simulink model "VehicleModel"  (R2020b)
settings: Solver=FixedStepAuto  StartTime=0.0  StopTime=1068  FixedStep=0.1  RelTol=1e-3
model workspace (MAT data in the model file):
  t = mpt.Parameter
  t.Value = 0
  t.DataType = 'auto'
  t.Dimensions = [1 1]
(part 1 of 5)
settings Model: Creator=User  LastModifiedBy=User

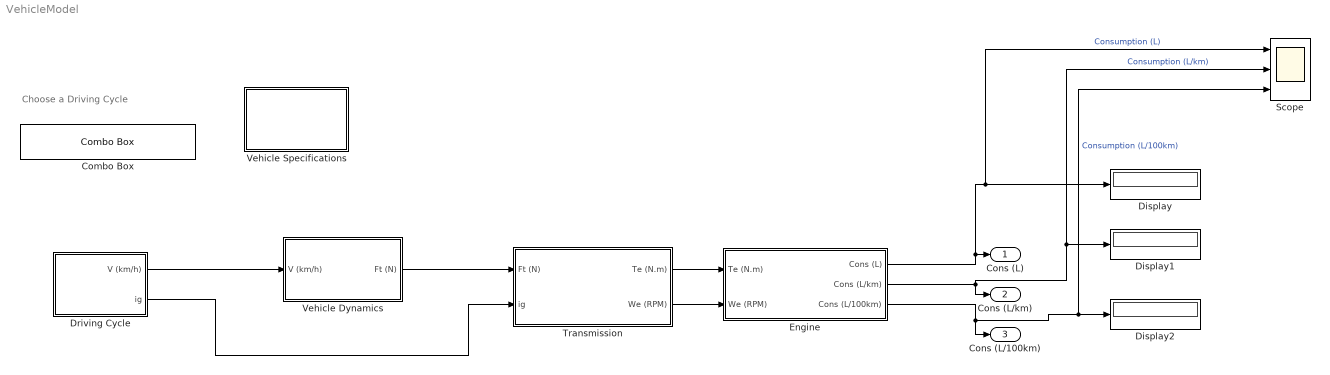
== system VehicleModel ==
  note: Choose a Driving Cycle
  Combo Box : ComboBox  LabelPosition=Hide  SelectedLabel=Highway
      settings: Values={{'Highway', 'Rural Road', 'Urban'}, [0 1 2]}
  Display : Display
  Display1 : Display
  Display2 : Display
  Driving Cycle : Subsystem
  Engine : Subsystem
  Scope : Scope  NumInputPorts=3
  Transmission : Subsystem
  Vehicle Dynamics : Subsystem
  Vehicle Specifications : Subsystem  mask{M=1320, g=9.81, rho=1.2, Af=2, Cx=0.3, rd=0.3, i0=3, ng=0.95, nd=0.97, dF=0.74, IdCon=1, IdSp=700}
      mask prompts: M "Vehicle Mass (kg)"; g "gravity (m/s2)"; rho "Air Density (kg/m3)"; Af "Surface Area (m2)"; Cx "Drag Coefficient"; rd "Dynamic Radius (m)"; i0 "Differential Gear Ratio"; ng "Gear Efficiency"; nd "Differential Efficiency"; dF "Fuel Density (kg/L)"; IdCon "Idle Consumption (L/h)"; IdSp "Idle Speed (RPM)"
  Cons (L) : Outport
  Cons (L/km) : Outport  Port=2
  Cons (L/100km) : Outport  Port=3
  wires:
  Vehicle Dynamics/1(Ft (N)) -> Transmission/1(Ft (N))
  Engine/1(Cons (L)) -> Scope/1, Display/1, Cons (L)/1  "Consumption (L)"
  Transmission/1(Te (N.m)) -> Engine/1(Te (N.m))
  Transmission/2(We (RPM)) -> Engine/2(We (RPM))
  Driving Cycle/1(" V (km/h)") -> Vehicle Dynamics/1(V (km/h))
  Engine/2(Cons (L/km)) -> Cons (L/km)/1, Scope/2, Display1/1  "Consumption (L/km)"
  Engine/3(Cons (L/100km)) -> Cons (L/100km)/1, Scope/3, Display2/1  "Consumption (L/100km)"
  Driving Cycle/2(ig) -> Transmission/2(ig)

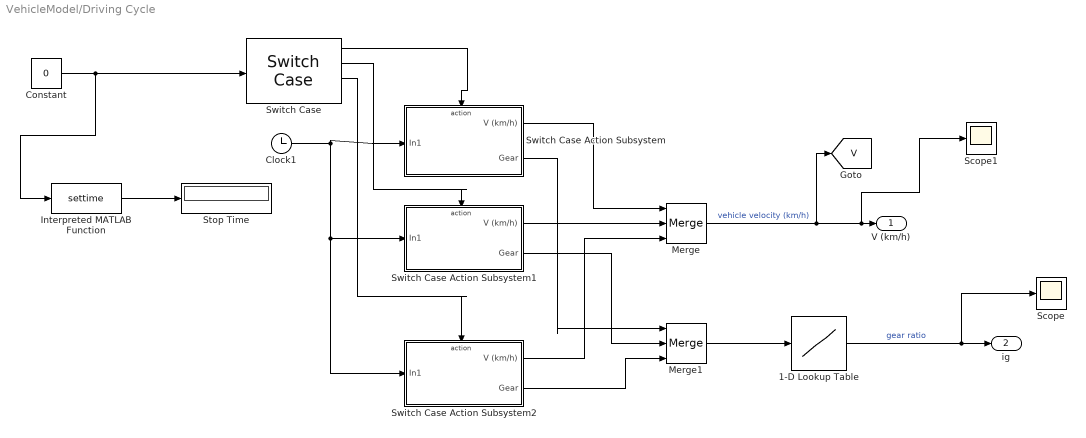
== system VehicleModel/Driving Cycle ==
  1-D Lookup Table : Lookup_n-D  NumberOfTableDimensions=1  BreakpointsForDimension1=[0 1 2 3 4 5]  Table=[0 3.5 2.31 1.52 1 0.66]  InternalRulePriority=Speed  RndMeth=Simplest  InputSameDT=on
  Clock1 : Clock
  Constant : Constant  Value=0
  Interpreted MATLAB Function : MATLABFcn  MATLABFcn=settime
  Merge : Merge  Inputs=3
  Merge1 : Merge  Inputs=3
  Scope : Scope
  Scope1 : Scope
  Stop Time : Display
  Switch Case : SwitchCase  CaseConditions={[0],[1],[2]}
  Switch Case Action Subsystem : Subsystem  TreatAsAtomicUnit=on
  Switch Case Action Subsystem1 : Subsystem  TreatAsAtomicUnit=on
  Switch Case Action Subsystem2 : Subsystem  TreatAsAtomicUnit=on
  " V (km/h)" : Outport
  ig : Outport  Port=2
  tag scope: V=global
  wires:
  1-D Lookup Table/1 -> Scope/1, ig/1  "gear ratio"
  Switch Case/1 -> Switch Case Action Subsystem/Action
  Clock1/1 -> Switch Case Action Subsystem/1(In1), Switch Case Action Subsystem1/1(In1), Switch Case Action Subsystem2/1(In1)
  Switch Case/2 -> Switch Case Action Subsystem1/Action
  Switch Case Action Subsystem1/1(V (km/h)) -> Merge/2
  Switch Case Action Subsystem/1(" V (km/h)") -> Merge/1
  Switch Case Action Subsystem/2(" Gear") -> Merge1/1
  Switch Case Action Subsystem1/2(Gear) -> Merge1/2
  Switch Case/3 -> Switch Case Action Subsystem2/Action
  Switch Case Action Subsystem2/1(V (km/h)) -> Merge/3
  Switch Case Action Subsystem2/2(Gear) -> Merge1/3
  Merge1/1 -> 1-D Lookup Table/1
  Merge/1 -> [V], Scope1/1, " V (km/h)"/1  "vehicle velocity (km/h)"
  Constant/1 -> Interpreted MATLAB Function/1, Switch Case/1
  Interpreted MATLAB Function/1 -> Stop Time/1

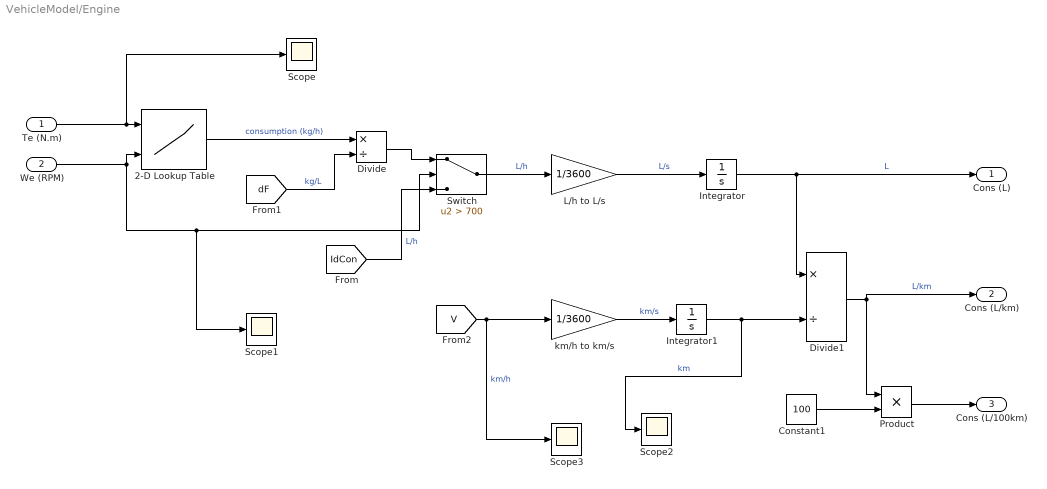
== system VehicleModel/Engine ==
  Te (N.m) : Inport
  We (RPM) : Inport  Port=2
  2-D Lookup Table : Lookup_n-D  BreakpointsForDimension1=|  BreakpointsForDimension2="[500\t1000\t1500\t2000\t2500\t3000\t3500\t4000\t4500\t5000\t5500\t6000]"  Table=|  InternalRulePriority=Speed  RndMeth=Simplest  InputSameDT=on
      BreakpointsForDimension1=|
      | [15.6
      | 31.2
      | 46.8
      | 62.4
      | 78
      | 93.6
      | 109.2
      | 124.8
      | 140.4
      | 156
      | 171.6]
      Table=|
      | [0.50	1.00	1.50	1.94	2.28	2.56	2.68	3.41	3.97	5.59	6.79	7.41;
      | 0.72	1.32	1.99	2.59	3.12	3.58	3.89	4.66	5.77	7.53	9.19	10.37;
      | 0.91	1.65	2.54	3.28	3.93	4.58	4.94	6.22	7.75	9.26	11.35	12.70;
      | 1.08	2.01	3.00	3.93	4.65	5.47	6.42	7.95	9.32	10.88	13.13	14.68;
      | 1.25	2.32	3.44	4.50	5.44	6.44	7.92	9.23	10.78	12.50	14.72	16.41;
      | 1.53	2.81	3.86	5.08	6.04	7.52	9.18	10.80	12.31	13.94	15.91	18.42;
      | 1.73	3.23	4.37	5.60	7.00	8.52	10.37	12.02	13.99	16.20	18.79	20.50;
      | 2.12	3.72	4.83	6.40	8.00	9.60	11.36	13.27	15.88	18.23	21.22	23.15;
      | 2.12	4.23	5.56	7.30	9.00	10.80	12.78	15.46	18.05	20.80	23.58	25.72;
      | 2.35	4.70	7.06	8.59	10.44	12.70	15.03	17.41	20.25	23.23	26.04	28.23;
      | 2.59	5.18	7.76	10.35	12.94	15.53	18.11	20.70	23.29	25.88	28.46	31.05]
      settings: InputPortMap=u0,u1
  Constant1 : Constant  Value=100
  Divide : Product  Inputs=*/
  Divide1 : Product  Inputs=*/
  Integrator : Integrator
  Integrator1 : Integrator
  L/h to L/s : Gain  Gain=1/3600
  Product : Product
  Scope{,1..3} (4 alike) : Scope
  Switch : Switch  Criteria=u2 > Threshold  Threshold=700
  km/h to km/s : Gain  Gain=1/3600
  Cons (L) : Outport
  Cons (L/km) : Outport  Port=2
  Cons (L/100km) : Outport  Port=3
  wires:
  Te (N.m)/1 -> Scope/1, 2-D Lookup Table/1
  Switch/1 -> L/h to L/s/1  "L/h"
  We (RPM)/1 -> 2-D Lookup Table/2, Scope1/1, Switch/2
  [dF] -> Divide/2  "kg/L"
  2-D Lookup Table/1 -> Divide/1  "consumption (kg/h)"
  L/h to L/s/1 -> Integrator/1  "L/s"
  [IdCon] -> Switch/3  "L/h"
  Integrator/1 -> Divide1/1, Cons (L)/1  "L"
  Divide/1 -> Switch/1
  [V] -> Scope3/1, km/h to km/s/1  "km/h"
  km/h to km/s/1 -> Integrator1/1  "km/s"
  Divide1/1 -> Cons (L/km)/1, Product/1  "L/km"
  Constant1/1 -> Product/2
  Product/1 -> Cons (L/100km)/1
  Integrator1/1 -> Scope2/1, Divide1/2  "km"

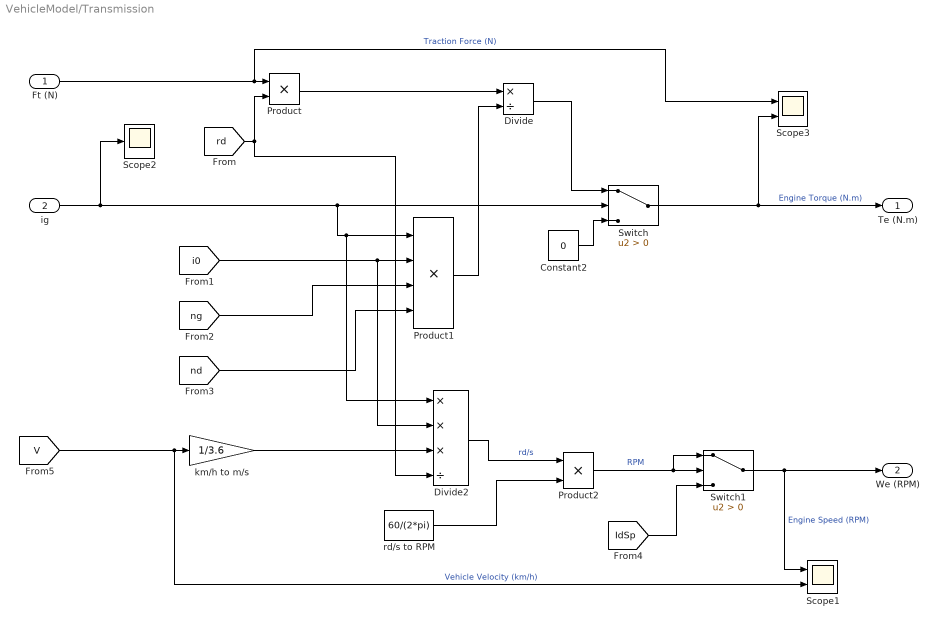
== system VehicleModel/Transmission ==
  Ft (N) : Inport
  ig : Inport  Port=2
  Constant2 : Constant  Value=0
  Divide : Product  Inputs=*/
  Divide2 : Product  Inputs=***/
  Product : Product
  Product1 : Product  Inputs=4
  Product2 : Product
  Scope1 : Scope  NumInputPorts=2
  Scope2 : Scope
  Scope3 : Scope  NumInputPorts=2
  Switch : Switch  Criteria=u2 > Threshold
  Switch1 : Switch  Criteria=u2 > Threshold
  km/h to m/s : Gain  Gain=1/3.6
  rd/s to RPM : Constant  Value=60/(2*pi)
  Te (N.m) : Outport
  We (RPM) : Outport  Port=2
  wires:
  Divide2/1 -> Product2/1  "rd/s"
  Product1/1 -> Divide/2
  rd/s to RPM/1 -> Product2/2
  Product/1 -> Divide/1
  ig/1 -> Switch/2, Divide2/1, Product1/1, Scope2/1
  [rd] -> Divide2/4, Product/2
  [i0] -> Divide2/2, Product1/2
  [ng] -> Product1/3
  Ft (N)/1 -> Scope3/1, Product/1  "Traction Force (N)"
  [nd] -> Product1/4
  Constant2/1 -> Switch/3
  Divide/1 -> Switch/1
  Switch/1 -> Scope3/2, Te (N.m)/1  "Engine Torque (N.m)"
  [V] -> Scope1/2, km/h to m/s/1  "Vehicle Velocity (km/h)"
  km/h to m/s/1 -> Divide2/3
  Product2/1 -> Switch1/2, Switch1/1  "RPM"
  Switch1/1 -> We (RPM)/1, Scope1/1  "Engine Speed (RPM)"
  [IdSp] -> Switch1/3

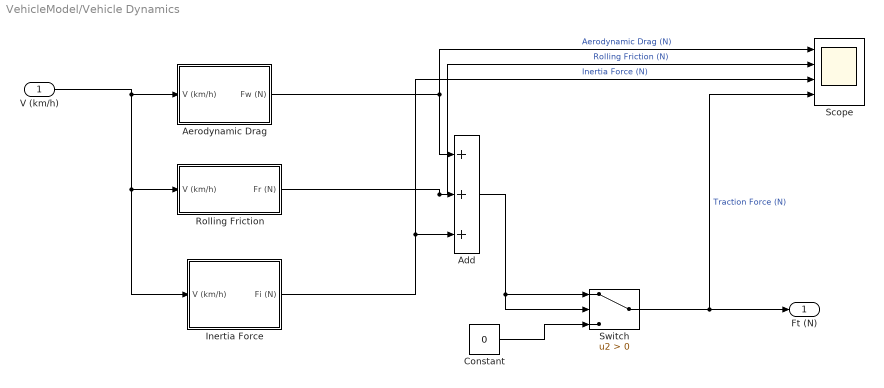
== system VehicleModel/Vehicle Dynamics ==
  V (km/h) : Inport
  Add : Sum  Inputs=+++
  Aerodynamic Drag : Subsystem
  Constant : Constant  Value=0
  Inertia Force : Subsystem
  Rolling Friction : Subsystem
  Scope : Scope  NumInputPorts=4
  Switch : Switch  Criteria=u2 > Threshold
  Ft (N) : Outport
  wires:
  V (km/h)/1 -> Aerodynamic Drag/1(V (km/h)), Rolling Friction/1(V (km/h)), Inertia Force/1(V (km/h))
  Aerodynamic Drag/1(Fw (N)) -> Add/1, Scope/1  "Aerodynamic Drag (N)"
  Rolling Friction/1(Fr (N)) -> Scope/2, Add/2  "Rolling Friction (N)"
  Inertia Force/1(Fi (N)) -> Add/3, Scope/3  "Inertia Force (N)"
  Add/1 -> Switch/2, Switch/1
  Constant/1 -> Switch/3
  Switch/1 -> Scope/4, Ft (N)/1  "Traction Force (N)"

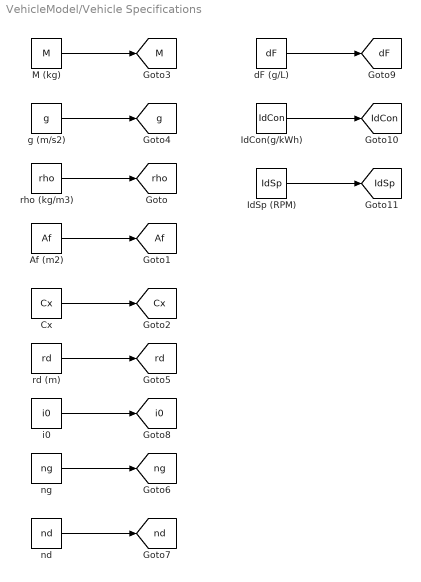
== system VehicleModel/Vehicle Specifications ==
  Af (m2) : Constant  Value=Af
  Cx : Constant  Value=Cx
  IdCon(g/kWh) : Constant  Value=IdCon
  IdSp (RPM) : Constant  Value=IdSp
  M (kg) : Constant  Value=M
  dF (g/L) : Constant  Value=dF
  g (m/s2) : Constant  Value=g
  i0 : Constant  Value=i0
  nd : Constant  Value=nd
  ng : Constant  Value=ng
  rd (m) : Constant  Value=rd
  rho (kg/m3) : Constant  Value=rho
  tag scope: Af=global, Cx=global, IdCon=global, IdSp=global, M=global, dF=global, g=global, i0=global, nd=global, ng=global, rd=global, rho=global
  wires:
  Cx/1 -> [Cx]
  Af (m2)/1 -> [Af]
  rho (kg/m3)/1 -> [rho]
  M (kg)/1 -> [M]
  g (m/s2)/1 -> [g]
  ng/1 -> [ng]
  nd/1 -> [nd]
  rd (m)/1 -> [rd]
  i0/1 -> [i0]
  IdCon(g/kWh)/1 -> [IdCon]
  dF (g/L)/1 -> [dF]
  IdSp (RPM)/1 -> [IdSp]
